simulink model "bpsk_symbol_level_transmission"  (R2026a)
settings: Solver=VariableStepAuto
model workspace (MAT data in the model file):
  FrameSize = 1000
  Tb = 0.001
libraries: commdigbbndpm3 x2, commchan3 x1, commrandsrc3 x1, commsink2 x1, commrflib2 x1
settings Model: Creator=ranja  LastModifiedBy=ranja

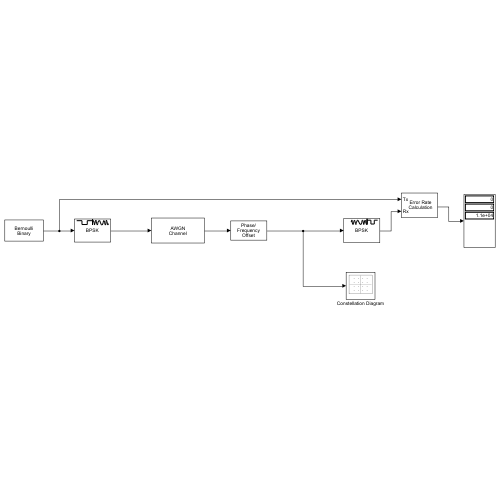
[thumbnail: Simulink's stored preview of the top-level diagram]
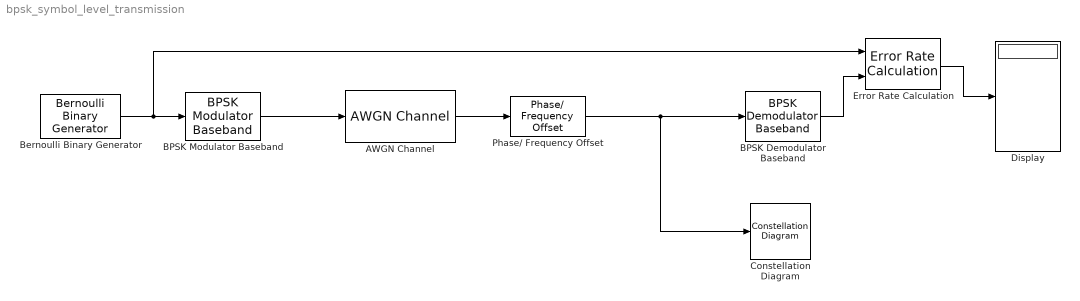
== system bpsk_symbol_level_transmission ==
  AWGN Channel : commchan3/AWGN Channel  LegacyMode=off  NoiseMethod="Signal to noise ratio  (SNR)"  noiseMode="Signal to noise ratio  (SNR)"  EbNo=10  EsNo=10  SNR=20  BitsPerSymbol=1  SignalPower=1  SpecifySymbolPeriod=off  SamplesPerSymbol=1  SymbolPeriod=1  VarianceSource=Parameter  Variance=1  RandomStream=Global stream  Seed=67  SimulateUsing=Code generation
  BPSK Demodulator Baseband : commdigbbndpm3/BPSK Demodulator Baseband  DecType=Hard decision  VarSource=Dialog  Variance=1  Ph=pi  outDtype=Inherit via internal rule  derotateFactorWordLen=16  derotateFactorDataTypeStr=Inherit: Same word length as input  derotateFactorLastDataTypeStr=Inherit: Same word length as input
      settings: LibrarySourceBlock=|
      | commhdldigbbndpm/BPSK
      | Demodulator
      | Baseband
  BPSK Modulator Baseband : commdigbbndpm3/BPSK Modulator Baseband  Ph=pi  outDtype=double  outWordLen=16  outUDDataType=sfix(16)  outFracLenMode=Best precision  outFracLen=15  outDataTypeStr=double  outLastDataTypeStr=double
      settings: LibrarySourceBlock=|
      | commhdldigbbndpm/BPSK
      | Modulator
      | Baseband
  Bernoulli Binary Generator : commrandsrc3/Bernoulli Binary Generator  ProbabilityOfZero=0.5  SeedSource=Auto  Seed=0  SampleTime=Tb  SamplesPerFrame=FrameSize  OutputDataType=double  SimulateUsing=Interpreted execution
  Constellation Diagram : ConstellationDiagram  WindowPosition=[1.000000,49.000000,1536.000000,793.000000,]  ScopeFrameLocation=window  ReferenceConstellation=BPSK  DefaultConfigurationName=comm.scopes.ConstellationDiagramBlockCfg
  Display : Display
  Error Rate Calculation : commsink2/Error Rate Calculation  N=0  st_delay=0  cp_mode=Entire frame  subframe=[]  PMode=Port  WsName=ErrorVec  RsMode2=off  stop=off  numErr=100  maxBits=1e6
      settings: LibrarySourceBlock=|
      | commhdlsink/Error Rate
      | Calculation
  Phase/ Frequency Offset : commrflib2/Phase// Frequency Offset  PhaseOffset=30  FrequencyOffsetFromPort=off  FrequencyOffset=0  SimulateUsing=Code generation
  wires:
  AWGN Channel/1 -> Phase/ Frequency Offset/1
  BPSK Demodulator Baseband/1 -> Error Rate Calculation/2
  Bernoulli Binary Generator/1 -> BPSK Modulator Baseband/1, Error Rate Calculation/1
  BPSK Modulator Baseband/1 -> AWGN Channel/1
  Error Rate Calculation/1 -> Display/1
  Phase/ Frequency Offset/1 -> Constellation Diagram/1, BPSK Demodulator Baseband/1
